simulink model "untitled"  (R2023b)
settings: Solver=VariableStepAuto  StartTime=0.0  StopTime=5000  RelTol=1e-3
values from neighbouring files (symbols this model uses):
  Cvl = Cp * rop * Vp    (= 150000)    [Lab1,1.m]    (also in Lab1.m; Lab1Wykres.m; Lab1gpt.m = 30000; WykresTempCzas.m = 30000)
  Cvp = Cp * rop * Vl    (= 30000)    [Lab1,1.m]    (also in Lab1.m; Lab1Wykres.m; Lab1gpt.m = 150000; WykresTempCzas.m = 150000)
  Ksl = a .* Ksp    [Lab1,1.m]    (also in Lab1.m = 173.913043478; Lab1Wykres.m = a * Ksp; Lab1gpt.m = 173.913043478; WykresTempCzas.m = 17.3913043478)
  Ksp = Pgn ./ (a .* (Tl - TzewN) + Tp - TzewN)    [Lab1,1.m]    (also in Lab1.m = 86.9565217391; Lab1Wykres.m = Pgn ./ (a * (Tl - TzewN) + Tp - TzewN); Lab1gpt.m = 86.9565217391; WykresTempCzas.m = 8.69565217391)
  Ksw = Ksp .* (Tp - TzewN) ./ (Tl - Tp)    [Lab1,1.m]    (also in Lab1.m = 608.695652174; Lab1Wykres.m = Ksp * (Tp - TzewN) / (Tl - Tp); Lab1gpt.m = 608.695652174; WykresTempCzas.m = 60.8695652174)
  Pg0 = Pgn+0    (= 10000)    [Lab1,1.m]    (also in Lab1.m; test.m)
  Tl_eq = double(sol.Tl_eq)    [Lab1Wykres.m]    (also in Lab1gpt.m = 20; WykresTempCzas.m = 20)
  Tp_eq = double(sol.Tp_eq)    [Lab1Wykres.m]    (also in Lab1gpt.m = 15; WykresTempCzas.m = 15)
  Tzew0 = TzewN+0    (= -20)    [Lab1,1.m]    (also in Lab1.m; test.m)
undefined symbols (not defined in the file or in its folder): dPg, dTzew
settings Model: Creator=pawli  LastModifiedBy=pawli

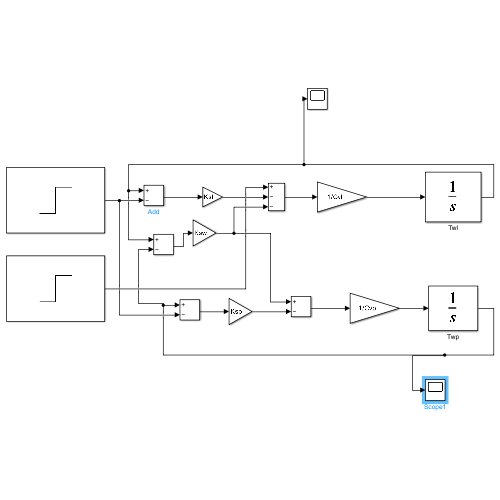
[thumbnail: Simulink's stored preview of the top-level diagram]
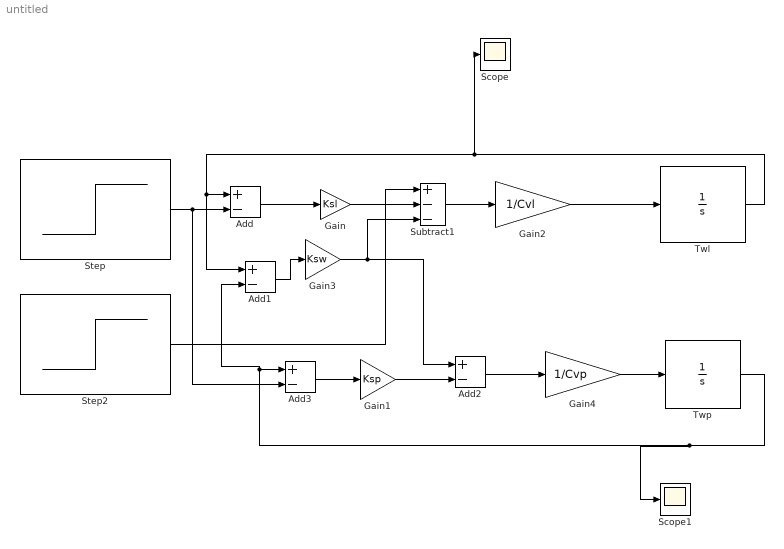
== system untitled ==
  Add{,1..3} (4 alike) : Sum  Inputs=+-
  Gain : Gain  Gain=Ksl
  Gain1 : Gain  Gain=Ksp
  Gain2 : Gain  Gain=1/Cvl
  Gain3 : Gain  Gain=Ksw
  Gain4 : Gain  Gain=1/Cvp
  Scope : Scope
  Scope1 : Scope
  Step : Step  Before=Tzew0  After=Tzew0+ dTzew  SampleTime=0
  Step2 : Step  Before=Pg0  After=Pg0 +dPg  SampleTime=0
  Subtract1 : Sum  Inputs=+--
  Twl : Integrator  InitialCondition=Tl_eq
  Twp : Integrator  InitialCondition=Tp_eq
  wires:
  Step/1 -> Add3/2, Add/2
  Add/1 -> Gain/1
  Gain/1 -> Subtract1/2
  Gain2/1 -> Twl/1
  Subtract1/1 -> Gain2/1
  Step2/1 -> Subtract1/1
  Gain3/1 -> Add2/1, Subtract1/3
  Add1/1 -> Gain3/1
  Gain4/1 -> Twp/1
  Add2/1 -> Gain4/1
  Add3/1 -> Gain1/1
  Gain1/1 -> Add2/2
  Twp/1 -> Scope1/1, Add3/1, Add1/2
  Twl/1 -> Scope/1, Add1/1, Add/1
